simulink model "helicoptertemplate"  (R2021b)
settings: Solver=ode45  StartTime=0.0  StopTime=T_tot  RelTol=1e-3
InitFcn:
  | hwinit
undefined symbols (not defined in the file or in its folder): adingain, adinoffs, h, HeliMexHandle
settings Model: Creator=fkzhang  LastModifiedBy=Dabbasi
settings SolverCC: AlgebraicLoopSolver=TrustRegion
settings DataIOCC: SaveFormat=Array  ReturnWorkspaceOutputs=off
settings OptimizationCC: BlockReduction=off  BooleanDataType=off  LifeSpan=inf
settings DebuggingCC: SaveWithParameterizedLinksMsg=none  UnderspecifiedInitializationDetection=Classic  MergeDetectMultiDrivingBlocksExec=none  SignalResolutionControl=TryResolveAllWithWarning  AllowSymbolicDim=off  SFUnexpectedBacktrackingDiag=warning  SFNoUnconditionalDefaultTransitionDiag=warning  SFExecutionAtInitializationDiag=none  SFMachineParentedDataDiag=warning  ArithmeticOperatorsInVariantConditions=warning
settings HardwareCC: ProdBitPerPointer=32  ProdBitPerSizeT=32  ProdBitPerPtrDiffT=32  ProdLargestAtomicFloat=None  ProdIntDivRoundTo=Undefined  ProdEndianess=Unspecified  ProdWordSize=32  ProdHWDeviceType=32-bit Generic  TargetUnknown=on
settings ModelReferenceCC: PropagateSignalLabelsOutOfModel=off
settings SFSimCC: SimUseLocalCustomCode=off  CustomCodeUndefinedFunction=UseInterfaceOnly
settings RTWCC: RTWUseLocalCustomCode=off
settings CodeAppCC: StateflowObjectComments=on
settings GRTTargetCC: TargetLangStandard=C89/C90 (ANSI)
settings ConfigComp: CovMetricSettings=dw  CovSaveCumulativeToWorkspaceVar=on  CovSaveSingleToWorkspaceVar=on  CovExternalEMLEnable=off  CovSFcnEnable=off

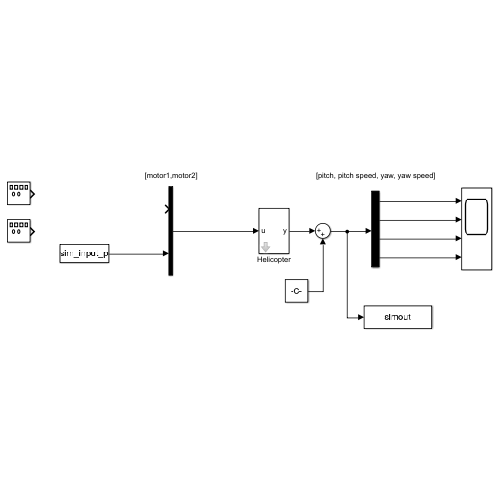
[thumbnail: Simulink's stored preview of the top-level diagram]
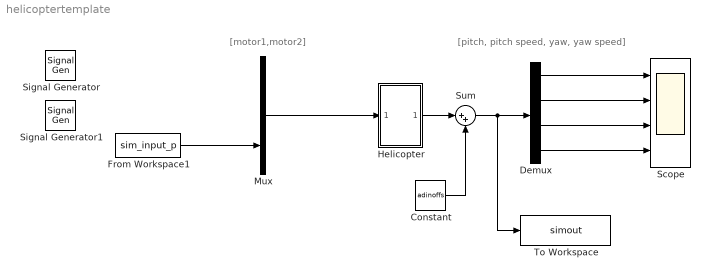
== system helicoptertemplate ==
  note: [pitch, pitch speed, yaw, yaw speed]
  note: [motor1,motor2]
  Constant : Constant  Value=adinoffs
  Demux : Demux
  From Workspace1 : FromWorkspace  VariableName=sim_input_p
  Helicopter : Subsystem  mask{Ts=h}
      mask prompts: Ts "sampletime"
      mask init:
      | sf_heli_init
      mask Display:
      | port_label('input',1,'u');
      | port_label('output',1,'y');
  Mux : Mux  Inputs=2
  Scope : Scope  NumInputPorts=4
  Signal Generator : SignalGenerator  WaveForm=square  Amplitude=0.6  Frequency=0.1
  Signal Generator1 : SignalGenerator  WaveForm=square  Amplitude=0  Frequency=0.8
  Sum : Sum  Inputs=|++
  To Workspace : ToWorkspace  VariableName=simout  SaveFormat=Timeseries  SampleTime=-1
  wires:
  Mux/1 -> Helicopter/1(In1)
  Demux/2 -> Scope/2
  Demux/3 -> Scope/3
  Demux/4 -> Scope/4
  Demux/1 -> Scope/1
  Helicopter/1(Out1) -> Sum/1
  Constant/1 -> Sum/2
  Sum/1 -> To Workspace/1, Demux/1
  From Workspace1/1 -> Mux/2

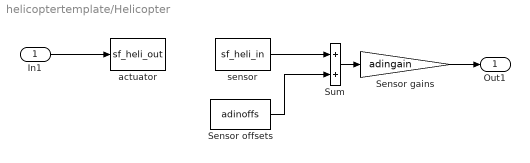
== system helicoptertemplate/Helicopter ==
  In1 : Inport
  Sensor gains : Gain  Gain=adingain
  Sensor offsets : Constant  Value=adinoffs
  Sum : Sum
  actuator : M-S-Function  FunctionName=sf_heli_out  Parameters=HeliMexHandle,Ts
  sensor : M-S-Function  FunctionName=sf_heli_in  Parameters=HeliMexHandle
  Out1 : Outport
  wires:
  sensor/1 -> Sum/1
  In1/1 -> actuator/1
  Sensor offsets/1 -> Sum/2
  Sum/1 -> Sensor gains/1
  Sensor gains/1 -> Out1/1
